simulink model "wheel_loader"  (R2026a)
settings: configuration reference "standardSILConfiguraitonParams" (kept outside this file)
undefined symbols (not defined in the file): vehicleParams
settings Model: Creator=jerem  LastModifiedBy=Edison Altamirano
settings ConfigSetRef: SourceName=standardSILConfiguraitonParams  SourceLocation=Base Workspace

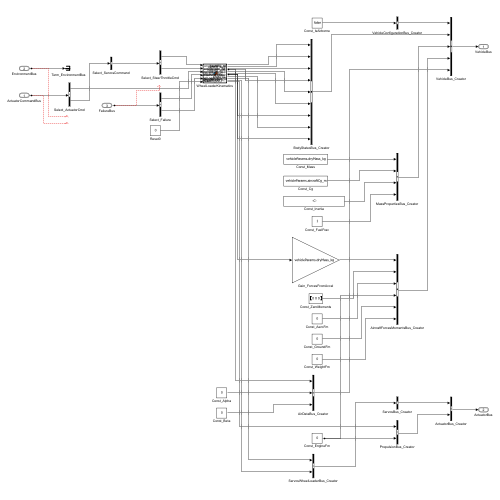
[thumbnail: Simulink's stored preview of the top-level diagram]
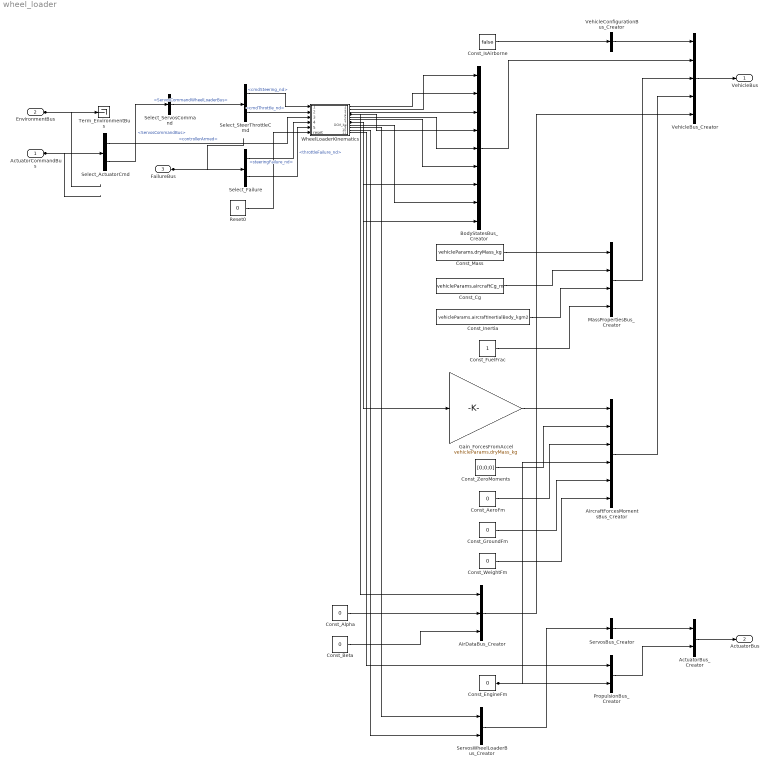
== system wheel_loader ==
  ActuatorCommandBus : Inport  OutDataTypeStr=Bus: ActuatorCommandBus
  EnvironmentBus : Inport  Port=2  OutDataTypeStr=Bus: EnvironmentBus
  FailureBus : Inport  Port=3  OutDataTypeStr=Bus: FailureBus
  ActuatorBus_Creator : BusCreator  Inputs=2  OutDataTypeStr=Bus: ActuatorBus
  AirDataBus_Creator : BusCreator  Inputs=3  OutDataTypeStr=Bus: AirDataBus
  AircraftForcesMomentsBus_Creator : BusCreator  Inputs=6  OutDataTypeStr=Bus: AircraftForcesMomentsBus
  BodyStatesBus_Creator : BusCreator  Inputs=9  OutDataTypeStr=Bus: BodyStateBus
  Const_AeroFm : Constant  Value=0  OutDataTypeStr=Bus: ComponentForcesMomentsBus
  Const_Alpha : Constant  Value=0
  Const_Beta : Constant  Value=0
  Const_Cg : Constant  Value=vehicleParams.aircraftCg_m
  Const_EngineFm : Constant  Value=0  OutDataTypeStr=Bus: ComponentForcesMomentsBus
  Const_FuelFrac : Constant
  Const_GroundFm : Constant  Value=0  OutDataTypeStr=Bus: ComponentForcesMomentsBus
  Const_Inertia : Constant  Value=vehicleParams.aircraftInertialBody_kgm2
  Const_IsAirborne : Constant  Value=false  OutDataTypeStr=boolean
  Const_Mass : Constant  Value=vehicleParams.dryMass_kg
  Const_WeightFm : Constant  Value=0  OutDataTypeStr=Bus: ComponentForcesMomentsBus
  Const_ZeroMoments : Constant  Value=[0;0;0]
  Gain_ForcesFromAccel : Gain  Gain=vehicleParams.dryMass_kg
  MassPropertiesBus_Creator : BusCreator  Inputs=4  OutDataTypeStr=Bus: MassPropertiesBus
  PropulsionBus_Creator : BusCreator  Inputs=2  OutDataTypeStr=Bus: PropulsionBus
  Reset0 : Constant  Value=0
  Select_ActuatorCmd : BusSelector  OutputSignals=controllerArmed,ServosCommandBus
  Select_Failure : BusSelector  OutputSignals=steeringFailure_nd,throttleFailure_nd
  Select_ServosCommand : BusSelector  OutputSignals=ServosCommandWheelLoaderBus
  Select_SteerThrottleCmd : BusSelector  OutputSignals=cmdSteering_nd,cmdThrottle_nd
  ServosBus_Creator : BusCreator  Inputs=1  OutDataTypeStr=Bus: ServosBus
  ServosWheelLoaderBus_Creator : BusCreator  Inputs=2  OutDataTypeStr=Bus: ServosWheelLoaderBus
  Term_EnvironmentBus : Terminator
  VehicleBus_Creator : BusCreator  Inputs=5  OutDataTypeStr=Bus: VehicleBus
  VehicleConfigurationBus_Creator : BusCreator  Inputs=1  OutDataTypeStr=Bus: VehicleConfigurationBus
  WheelLoaderKinematics : MATLAB Function  TreatAsAtomicUnit=on
  VehicleBus : Outport  OutDataTypeStr=Bus: VehicleBus
  ActuatorBus : Outport  Port=2  OutDataTypeStr=Bus: ActuatorBus
  wires:
  EnvironmentBus/1 -> Term_EnvironmentBus/1
  PropulsionBus_Creator/1 -> ActuatorBus_Creator/2
  Const_ZeroMoments/1 -> AircraftForcesMomentsBus_Creator/2
  FailureBus/1 -> Select_Failure/1
  ActuatorCommandBus/1 -> Select_ActuatorCmd/1
  BodyStatesBus_Creator/1 -> VehicleBus_Creator/2
  Select_ActuatorCmd/1 -> WheelLoaderKinematics/3(controllerArmed)  "<controllerArmed>"
  Select_SteerThrottleCmd/2 -> WheelLoaderKinematics/2(cmdThrottle_nd)  "<cmdThrottle_nd>"
  Select_SteerThrottleCmd/1 -> WheelLoaderKinematics/1(cmdSteering_nd)  "<cmdSteering_nd>"
  Select_ServosCommand/1 -> Select_SteerThrottleCmd/1  "<ServosCommandWheelLoaderBus>"
  Const_Mass/1 -> MassPropertiesBus_Creator/1
  Select_ActuatorCmd/2 -> Select_ServosCommand/1  "<ServosCommandBus>"
  Select_Failure/1 -> WheelLoaderKinematics/4(steeringFailure_nd)  "<steeringFailure_nd>"
  WheelLoaderKinematics/8(DCM_be) -> BodyStatesBus_Creator/8
  Reset0/1 -> WheelLoaderKinematics/6(reset)
  Select_Failure/2 -> WheelLoaderKinematics/5(throttleFailure_nd)  "<throttleFailure_nd>"
  AirDataBus_Creator/1 -> VehicleBus_Creator/5
  WheelLoaderKinematics/1(posNED_m) -> BodyStatesBus_Creator/2
  WheelLoaderKinematics/2(velNED_mps) -> BodyStatesBus_Creator/1
  VehicleConfigurationBus_Creator/1 -> VehicleBus_Creator/1
  WheelLoaderKinematics/3(eulerAngles_rad) -> BodyStatesBus_Creator/3
  WheelLoaderKinematics/4(velBody_mps) -> BodyStatesBus_Creator/4, AirDataBus_Creator/1
  ServosWheelLoaderBus_Creator/1 -> ServosBus_Creator/1
  WheelLoaderKinematics/5(angVelBody_radps) -> BodyStatesBus_Creator/5
  WheelLoaderKinematics/6(angAccelBody_radps2) -> BodyStatesBus_Creator/6
  WheelLoaderKinematics/7(accelBody_mps2) -> BodyStatesBus_Creator/7, BodyStatesBus_Creator/9, Gain_ForcesFromAccel/1
  WheelLoaderKinematics/9(steeringAngle_rad) -> ServosWheelLoaderBus_Creator/1
  WheelLoaderKinematics/10(wheelSpeed_radps) -> ServosWheelLoaderBus_Creator/2
  WheelLoaderKinematics/11(motorAngVel_radps) -> PropulsionBus_Creator/1
  Const_Alpha/1 -> AirDataBus_Creator/2
  Const_Cg/1 -> MassPropertiesBus_Creator/2
  Const_Beta/1 -> AirDataBus_Creator/3
  Const_IsAirborne/1 -> VehicleConfigurationBus_Creator/1
  AircraftForcesMomentsBus_Creator/1 -> VehicleBus_Creator/4
  Const_Inertia/1 -> MassPropertiesBus_Creator/3
  Const_FuelFrac/1 -> MassPropertiesBus_Creator/4
  VehicleBus_Creator/1 -> VehicleBus/1
  Gain_ForcesFromAccel/1 -> AircraftForcesMomentsBus_Creator/1
  Const_AeroFm/1 -> AircraftForcesMomentsBus_Creator/3
  Const_GroundFm/1 -> AircraftForcesMomentsBus_Creator/5
  Const_WeightFm/1 -> AircraftForcesMomentsBus_Creator/6
  ActuatorBus_Creator/1 -> ActuatorBus/1
  Const_EngineFm/1 -> PropulsionBus_Creator/2, AircraftForcesMomentsBus_Creator/4
  MassPropertiesBus_Creator/1 -> VehicleBus_Creator/3
  ServosBus_Creator/1 -> ActuatorBus_Creator/1

== matlab function wheel_loader/WheelLoaderKinematics ==
  data: cmdSteering_nd input; posNED_m output; cmdThrottle_nd input; controllerArmed input; steeringFailure_nd input; throttleFailure_nd input; reset input; velNED_mps output; eulerAngles_rad output; velBody_mps output; angVelBody_radps output; angAccelBody_radps2 output; accelBody_mps2 output; DCM_be output; steeringAngle_rad output; wheelSpeed_radps output; motorAngVel_radps output
function [posNED_m, velNED_mps, eulerAngles_rad, velBody_mps, angVelBody_radps, angAccelBody_radps2, accelBody_mps2, DCM_be, steeringAngle_rad, wheelSpeed_radps, motorAngVel_radps] = WheelLoaderKinematics(cmdSteering_nd, cmdThrottle_nd, controllerArmed, steeringFailure_nd, throttleFailure_nd, reset)
%#codegen
persistent posN posE yaw speed steerAngle
if isempty(posN) || reset
    posN = 0; posE = 0; yaw = 1.9199; speed = 0; steerAngle = 0;
end
Ts = 0.004;
wheelBase_m = 2.5;
wheelRadius_m = 0.6;
maxSteerAngle_rad = 0.5;
maxSpeed_mps = 4.0;
tauSteer_s = 0.4;
tauThrottle_s = 0.8;
referenceAltitude_m = 116 * 0.3048;
if steeringFailure_nd
    steerCmd_rad = steerAngle;
else
    steerCmd_rad = cmdSteering_nd * maxSteerAngle_rad;
end
if throttleFailure_nd || ~controllerArmed
    speedCmd_mps = 0;
else
    speedCmd_mps = cmdThrottle_nd * maxSpeed_mps;
end
speedDot = (speedCmd_mps - speed) / tauThrottle_s;
yawRate = speed / wheelBase_m * tan(steerAngle);
posN = posN + Ts * speed * cos(yaw);
posE = posE + Ts * speed * sin(yaw);
yaw = yaw + Ts * yawRate;
speed = speed + Ts * speedDot;
steerAngle = steerAngle + Ts * (steerCmd_rad - steerAngle) / tauSteer_s;
posNED_m = [posN; posE; -referenceAltitude_m];
velNED_mps = [speed*cos(yaw); speed*sin(yaw); 0];
eulerAngles_rad = [0; 0; yaw];
velBody_mps = [speed; 0; 0];
angVelBody_radps = [0; 0; yawRate];
angAccelBody_radps2 = [0; 0; 0];
accelBody_mps2 = [speedDot; speed*yawRate; 0];
DCM_be = [cos(yaw) sin(yaw) 0; -sin(yaw) cos(yaw) 0; 0 0 1];
steeringAngle_rad = steerAngle;
wheelSpeed_radps = speed / wheelRadius_m;
motorAngVel_radps = wheelSpeed_radps;
